simulink model "Hotendcontrol"  (R2025b)
settings: Solver=VariableStepAuto  StartTime=0.0  StopTime=10.0  RelTol=1e-3
undefined symbols (not defined in the file or in its folder): A, B, C, K_motor, Nbar_motor
settings Model: Creator=kenom  LastModifiedBy=kenom

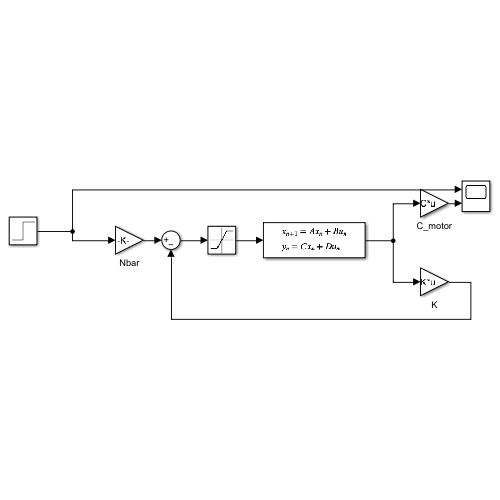
[thumbnail: Simulink's stored preview of the top-level diagram]
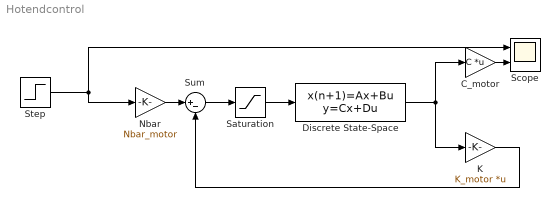
== system Hotendcontrol ==
  C_motor : Gain  Gain=C  Multiplication=Matrix(K*u)
  Discrete State-Space : DiscreteStateSpace  A=A  B=B  C=eye(size(A))  D=zeros(size(A,1),1)  SampleTime=0.1
  K : Gain  Gain=K_motor  Multiplication=Matrix(K*u)
  Nbar : Gain  Gain=Nbar_motor
  Saturation : Saturate  UpperLimit=255  LowerLimit=-255
  Scope : Scope  NumInputPorts=2
      settings: ActiveDisplayYMinimum=-4.3945210994805537  ActiveDisplayYMaximum=39.550689895324993
  Step : Step  After=35  SampleTime=0
  Sum : Sum  Inputs=|+-
  wires:
  Nbar/1 -> Sum/1
  Sum/1 -> Saturation/1
  Saturation/1 -> Discrete State-Space/1
  K/1 -> Sum/2
  Step/1 -> Nbar/1, Scope/1
  Discrete State-Space/1 -> C_motor/1, K/1
  C_motor/1 -> Scope/2
